simulink model "chap3_1sim"  (Simulink 7.7)
settings: Solver=ode45  StartTime=0.0  StopTime=30  RelTol=1e-3
settings Model: Creator=ljk  LastModifiedBy=ljk  ExtModeTrigMode=oneshot  ExtModeArmWhenConnect=off
settings DataIOCC: Decimation=100  LimitDataPoints=off  SaveOutput=off  SaveTime=off  SignalLoggingName=sigsOut
settings OptimizationCC: BooleanDataType=off
settings DebuggingCC: SaveWithParameterizedLinksMsg=none  SignalResolutionControl=TryResolveAllWithWarning  SolverPrmCheckMsg=none  MultiTaskDSMMsg=warning  MultiTaskCondExecSysMsg=none  StrictBusMsg=None
settings HardwareCC: TargetUnknown=on
settings RTWCC: IncludeERTFirstTime=on

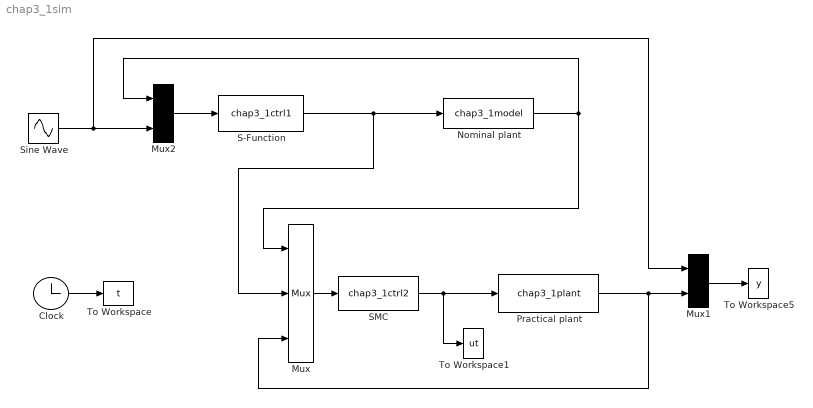
== system chap3_1sim ==
  Clock : Clock
  Mux : Mux  Inputs=3
  Mux1 : Mux  Inputs=2
  Mux2 : Mux  Inputs=2
  Nominal plant : S-Function  FunctionName=chap3_1model  EnableBusSupport=off
  Practical plant : S-Function  FunctionName=chap3_1plant  EnableBusSupport=off
  S-Function : S-Function  FunctionName=chap3_1ctrl1  EnableBusSupport=off
  SMC : S-Function  FunctionName=chap3_1ctrl2  EnableBusSupport=off
  Sine Wave : Sin  SampleTime=0
  To Workspace : ToWorkspace  VariableName=t  SampleTime=-1  SaveFormat=Array
  To Workspace1 : ToWorkspace  VariableName=ut  SampleTime=-1  SaveFormat=Array
  To Workspace5 : ToWorkspace  VariableName=y  SampleTime=-1  SaveFormat=Array
  wires:
  Clock/1 -> To Workspace/1
  Mux/1 -> SMC/1
  SMC/1 -> Practical plant/1, To Workspace1/1
  Sine Wave/1 -> Mux2/2, Mux1/1
  Mux2/1 -> S-Function/1
  Mux1/1 -> To Workspace5/1
  Practical plant/1 -> Mux/3, Mux1/2
  Nominal plant/1 -> Mux2/1, Mux/1
  S-Function/1 -> Nominal plant/1, Mux/2
